simulink model "Problem_4"  (R2020b)
settings: Solver=VariableStepAuto  StartTime=0.0  StopTime=10.0  RelTol=1e-3
settings Model: Creator=HP  LastModifiedBy=HP

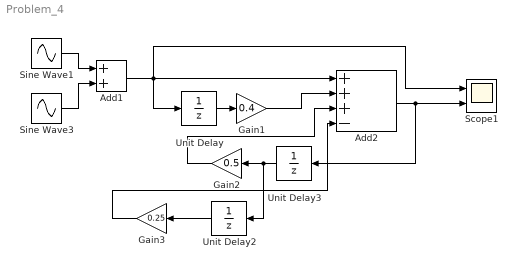
== system Problem_4 ==
  Add1 : Sum
  Add2 : Sum  Inputs=+++-
  Gain1 : Gain  Gain=0.4
  Gain2 : Gain  Gain=0.5
  Gain3 : Gain  Gain=0.25
  Scope1 : Scope  NumInputPorts=2
  Sine Wave1 : Sin  SampleTime=0
  Sine Wave3 : Sin  Amplitude=0.5  Frequency=50  SampleTime=0
  Unit Delay : UnitDelay  SampleTime=-1  HasFrameUpgradeWarning=on
  Unit Delay2 : UnitDelay  SampleTime=-1  HasFrameUpgradeWarning=on
  Unit Delay3 : UnitDelay  SampleTime=-1  HasFrameUpgradeWarning=on
  wires:
  Gain1/1 -> Add2/2
  Add2/1 -> Unit Delay3/1, Scope1/2
  Add1/1 -> Add2/1, Scope1/1, Unit Delay/1
  Unit Delay/1 -> Gain1/1
  Unit Delay2/1 -> Gain3/1
  Sine Wave1/1 -> Add1/1
  Gain2/1 -> Add2/3
  Unit Delay3/1 -> Unit Delay2/1, Gain2/1
  Gain3/1 -> Add2/4
  Sine Wave3/1 -> Add1/2
